simulink model "Diagram"  (R2019a)
settings: Solver=VariableStepAuto  StartTime=0.0  StopTime=10.0  RelTol=1e-3
undefined symbols (not defined in the file): fdesignblkfcn, gcbh
libraries: dspxfrm3 x1, simulink_extras x1, ec_arm_cortex_a_lib x1
settings Model: Creator=bamba  LastModifiedBy=bamba

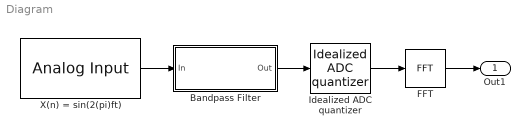
== system Diagram ==
  Bandpass Filter : Subsystem  DialogController=fdesignblkfcn  InitFcn=fdesignblkfcn(gcbh, {'InitFcn'});  mask(Bandpass Filter){}
      mask help: Design a bandpass filter
      settings: CopyFcn=fdesignblkfcn(gcbh, {'CopyFcn'});
      mask Help: helpview(mapfilelocation('dsp'), 'dspbandpassfilter');
      mask Display: disp('Bandpass');
  FFT : dspxfrm3/FFT  FFTImplementation=Auto  CompMethod=Table lookup  TableOpt=NEW  TableOptActive=Speed  BitRevOrder=off  Normalize=off  InheritFFTLength=on  FFTLength=64  WrapInput=on  roundingMode=Floor  overflowMode=off  firstCoeffDataTypeStr=Inherit: Same word length as input  firstCoeffLastDataTypeStr=Inherit: Same word length as input  outputMin=[]  outputMax=[]
  Idealized ADC quantizer : simulink_extras/Additional Discrete/Idealized ADC quantizer  NumberOfConverterBits=12  Vmin=0  Vmax=5  OutputDataType=int16  OutputNegativeValues=off
      settings: SourceProductName=Simulink
  X(n) = sin(2(pi)ft) : ec_arm_cortex_a_lib/Analog Input  board=BeagleBone Black  pin=P9_39  sampleTime=0.1  blockPlatform=BeagleBone
      settings: SourceProductName=Embedded Coder Support Package for ARM Cortex-A Processors  SourceProductBaseCode=ECCORTEXA
  Out1 : Outport  SignalName=X(m)
  wires:
  Bandpass Filter/1(Out) -> Idealized ADC quantizer/1
  FFT/1 -> Out1/1
  Idealized ADC quantizer/1 -> FFT/1
  X(n) = sin(2(pi)ft)/1 -> Bandpass Filter/1(In)

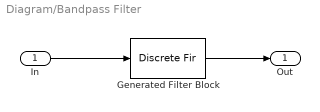
== system Diagram/Bandpass Filter ==
  In : Inport
  Generated Filter Block : DiscreteFir  Tag=BlockMethodSubSystem  Coefficients=[-0.0008992291487744296 0.0016414518747943749 0.0031352071842225397 -0.0040707550828814922 -0.0063731852227904111 0.0074874286806090491 0.0098354319566295711 -0.010189316513446216 -0.011302794465874122 0.0096929185841818435 0.0079428653987464216 -0.0031368247881221642 0.0028299878877943137 -0.011508674243001471 -0.022080136219461581 0.034245325424507672 0.048356661648905473 -0.062355369169884239 -0.077503478162593897 0.090687768153125653 0.10353171105844157 -0.11297860084229834 -0.12035866024978455 0.12379360801539134 0.12379360801539134 -0.12035866024978455 -0.11297860084229834 0.10353171105844157 0.090687768153125653 -0.077503478162593897 -0.062355369169884239 0.048356661648905473 0.034245325424507672 -0.022080136219461581 -0.011508674243001471 0.0028299878877943137 -0.0031368247881221642 0.0079428653987464216 0.0096929185841818435 -0.011302794465874122 -0.010189316513446216 0.0098354319566295711 0.0074874286806090491 -0.0063731852227904111 -0.0040707550828814922 0.0031352071842225397 0.0016414518747943749 -0.0008992291487744296]  InputProcessing=Columns as channels (frame based)
  Out : Outport
  wires:
  In/1 -> Generated Filter Block/1
  Generated Filter Block/1 -> Out/1
